simulink model "dynamics"  (R2022a)
settings: Solver=VariableStepAuto  StartTime=0.0  StopTime=10.0  RelTol=1e-3
undefined symbols (not defined in the file): b, g, h, I, J, K, L, m, R, Res
libraries: slpidlib x3
settings Model: Creator=daixingze  LastModifiedBy=xngzdai
settings SolverCC: AlgebraicLoopSolver=TrustRegion
settings DebuggingCC: UnconnectedInputMsg=warning  UnconnectedOutputMsg=warning  UnconnectedLineMsg=warning  SFMachineParentedDataDiag=warning

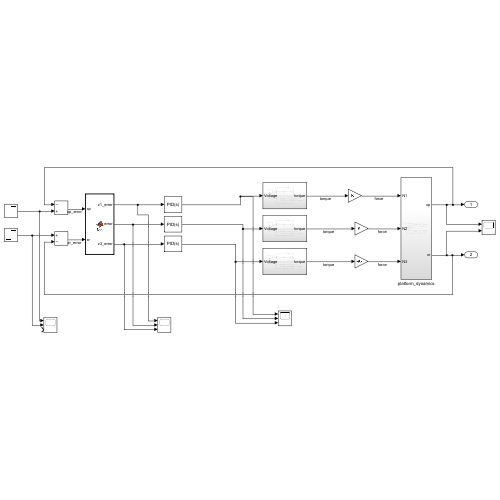
[thumbnail: Simulink's stored preview of the top-level diagram]
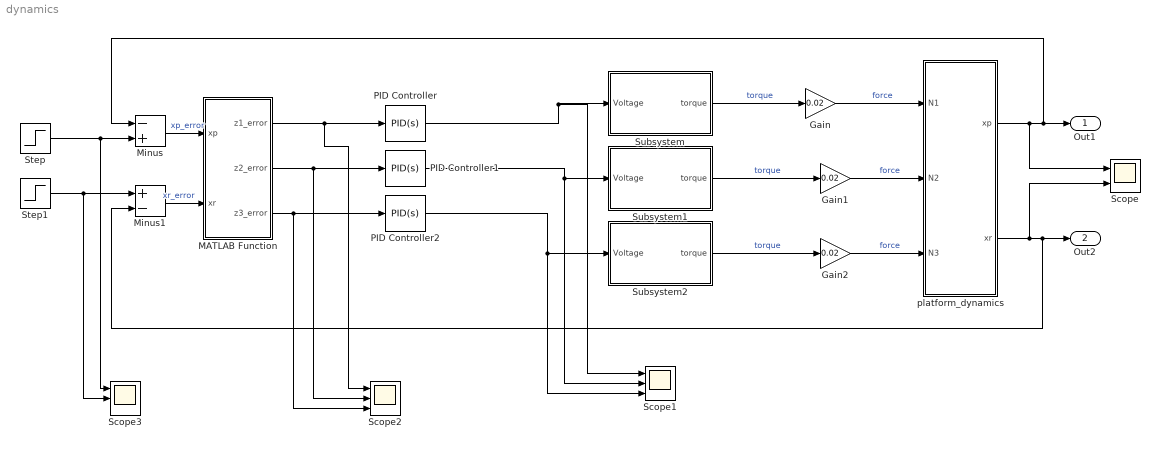
== system dynamics ==
  Gain : Gain  Gain=0.02
  Gain1 : Gain  Gain=0.02
  Gain2 : Gain  Gain=0.02
  MATLAB Function : MATLAB Function  TreatAsAtomicUnit=on
  Minus : Sum  Inputs=-+
  Minus1 : Sum  Inputs=+-
  PID Controller : slpidlib/PID Controller  Controller=PID  Form=Parallel  TimeDomain=Continuous-time  UseExternalTs=off  SampleTime=-1  IntegratorMethod=Forward Euler  FilterMethod=Forward Euler  ControllerParametersSource=internal  P=0.0002  I=0  UseKiTs=off  D=0.0000005  N=100  UseFilter=on  TunerSelectOption=Transfer Function Based (PID Tuner App)  InitialConditionSource=internal  InitialConditionForIntegrator=0  InitialConditionForFilter=0  DifferentiatorICPrevScaledInput=0  ExternalReset=none  TrackingMode=off  Kt=1  LimitOutput=off  SatLimitsSource=internal  UpperSaturationLimit=inf  LowerSaturationLimit=-inf  LinearizeAsGain=on  AntiWindupMode=none  Kb=1  POutMin=[]  POutMax=[]  IOutMin=[]  IOutMax=[]  DOutMin=[]  DOutMax=[]  NOutMin=[]  NOutMax=[]  SumOutMin=[]  SumOutMax=[]  SaturationOutMin=[]  SaturationOutMax=[]  PParamMin=[]  PParamMax=[]  IParamMin=[]  IParamMax=[]  DParamMin=[]  DParamMax=[]  NParamMin=[]  NParamMax=[]  KbParamMin=[]  KbParamMax=[]  KtParamMin=[]  KtParamMax=[]  KbOutMin=[]  KbOutMax=[]  KtOutMin=[]  KtOutMax=[]  IntegratorOutMin=[]  IntegratorOutMax=[]  FilterOutMin=[]  FilterOutMax=[]  SumI1OutMin=[]  SumI1OutMax=[]  SumI2OutMin=[]  SumI2OutMax=[]  SumI3OutMin=[]  SumI3OutMax=[]  SumI4OutMin=[]  SumI4OutMax=[]  SumDOutMin=[]  SumDOutMax=[]  DifferentiatorOutMin=[]  DifferentiatorOutMax=[]  FilterDiffOutCoefMin=[]  FilterDiffOutCoefMax=[]  ReciprocalOutMin=[]  ReciprocalOutMax=[]  SumDenOutMin=[]  SumDenOutMax=[]  SumNumOutMin=[]  SumNumOutMax=[]  DivideOutMin=[]  DivideOutMax=[]  UdiffTsProdOutMin=[]  UdiffTsProdOutMax=[]  NTsProdOutMin=[]  NTsProdOutMax=[]  UintegralTsProdOutMin=[]  UintegralTsProdOutMax=[]  UngainTsProdOutMin=[]  UngainTsProdOutMax=[]  IntegratorContinuousStateAttributes=''  IntegratorStateMustResolveToSignalObject=off  IntegratorRTWStateStorageClass=Auto  FilterContinuousStateAttributes=''  FilterStateMustResolveToSignalObject=off  FilterRTWStateStorageClass=Auto  ParallelPVariant=InternalParameters  IdealPVariant=Disabled  IVariant=InternalParameters  DVariant=InternalParameters  IntegratorVariant=Continuous  SatVariant=Disabled  AWVariant=Passthrough  PCopyVariant=Disabled  TRVariant=Disabled  FdbkBlocksVariant=Forward  IdealPFdbkVariant=Disabled  SatFdbkVariant=Disabled  DerivativeFilterVariant=ContFilter  NVariant=InternalParameters  NCopyVariant=Disabled  FilterICVariant=InternalICsFilter  IntegratorICVariant=InternalICs  ExternalResetVariant=Disabled  TRSumVariant=Passthrough  SumFdbkVariant=Disabled  SumVariant=Sum_PID  TsampFilterVariant=InternalTs  TsampNgainVariant=Passthrough  TsampIntegralVariant=Passthrough  ExternalSaturationOutDataTypeStr=Inherit: Same as second input  aMode=0
  PID Controller1 : slpidlib/PID Controller  Controller=PID  Form=Parallel  TimeDomain=Continuous-time  UseExternalTs=off  SampleTime=-1  IntegratorMethod=Forward Euler  FilterMethod=Forward Euler  ControllerParametersSource=internal  P=0.0002  I=0  UseKiTs=off  D=0.0000005  N=100  UseFilter=on  TunerSelectOption=Transfer Function Based (PID Tuner App)  InitialConditionSource=internal  InitialConditionForIntegrator=0  InitialConditionForFilter=0  DifferentiatorICPrevScaledInput=0  ExternalReset=none  TrackingMode=off  Kt=1  LimitOutput=off  SatLimitsSource=internal  UpperSaturationLimit=inf  LowerSaturationLimit=-inf  LinearizeAsGain=on  AntiWindupMode=none  Kb=1  POutMin=[]  POutMax=[]  IOutMin=[]  IOutMax=[]  DOutMin=[]  DOutMax=[]  NOutMin=[]  NOutMax=[]  SumOutMin=[]  SumOutMax=[]  SaturationOutMin=[]  SaturationOutMax=[]  PParamMin=[]  PParamMax=[]  IParamMin=[]  IParamMax=[]  DParamMin=[]  DParamMax=[]  NParamMin=[]  NParamMax=[]  KbParamMin=[]  KbParamMax=[]  KtParamMin=[]  KtParamMax=[]  KbOutMin=[]  KbOutMax=[]  KtOutMin=[]  KtOutMax=[]  IntegratorOutMin=[]  IntegratorOutMax=[]  FilterOutMin=[]  FilterOutMax=[]  SumI1OutMin=[]  SumI1OutMax=[]  SumI2OutMin=[]  SumI2OutMax=[]  SumI3OutMin=[]  SumI3OutMax=[]  SumI4OutMin=[]  SumI4OutMax=[]  SumDOutMin=[]  SumDOutMax=[]  DifferentiatorOutMin=[]  DifferentiatorOutMax=[]  FilterDiffOutCoefMin=[]  FilterDiffOutCoefMax=[]  ReciprocalOutMin=[]  ReciprocalOutMax=[]  SumDenOutMin=[]  SumDenOutMax=[]  SumNumOutMin=[]  SumNumOutMax=[]  DivideOutMin=[]  DivideOutMax=[]  UdiffTsProdOutMin=[]  UdiffTsProdOutMax=[]  NTsProdOutMin=[]  NTsProdOutMax=[]  UintegralTsProdOutMin=[]  UintegralTsProdOutMax=[]  UngainTsProdOutMin=[]  UngainTsProdOutMax=[]  IntegratorContinuousStateAttributes=''  IntegratorStateMustResolveToSignalObject=off  IntegratorRTWStateStorageClass=Auto  FilterContinuousStateAttributes=''  FilterStateMustResolveToSignalObject=off  FilterRTWStateStorageClass=Auto  ParallelPVariant=InternalParameters  IdealPVariant=Disabled  IVariant=InternalParameters  DVariant=InternalParameters  IntegratorVariant=Continuous  SatVariant=Disabled  AWVariant=Passthrough  PCopyVariant=Disabled  TRVariant=Disabled  FdbkBlocksVariant=Forward  IdealPFdbkVariant=Disabled  SatFdbkVariant=Disabled  DerivativeFilterVariant=ContFilter  NVariant=InternalParameters  NCopyVariant=Disabled  FilterICVariant=InternalICsFilter  IntegratorICVariant=InternalICs  ExternalResetVariant=Disabled  TRSumVariant=Passthrough  SumFdbkVariant=Disabled  SumVariant=Sum_PID  TsampFilterVariant=InternalTs  TsampNgainVariant=Passthrough  TsampIntegralVariant=Passthrough  ExternalSaturationOutDataTypeStr=Inherit: Same as second input  aMode=0
  PID Controller2 : slpidlib/PID Controller  Controller=PID  Form=Parallel  TimeDomain=Continuous-time  UseExternalTs=off  SampleTime=-1  IntegratorMethod=Forward Euler  FilterMethod=Forward Euler  ControllerParametersSource=internal  P=0.0002  I=0  UseKiTs=off  D=0.0000005  N=100  UseFilter=on  TunerSelectOption=Transfer Function Based (PID Tuner App)  InitialConditionSource=internal  InitialConditionForIntegrator=0  InitialConditionForFilter=0  DifferentiatorICPrevScaledInput=0  ExternalReset=none  TrackingMode=off  Kt=1  LimitOutput=off  SatLimitsSource=internal  UpperSaturationLimit=inf  LowerSaturationLimit=-inf  LinearizeAsGain=on  AntiWindupMode=none  Kb=1  POutMin=[]  POutMax=[]  IOutMin=[]  IOutMax=[]  DOutMin=[]  DOutMax=[]  NOutMin=[]  NOutMax=[]  SumOutMin=[]  SumOutMax=[]  SaturationOutMin=[]  SaturationOutMax=[]  PParamMin=[]  PParamMax=[]  IParamMin=[]  IParamMax=[]  DParamMin=[]  DParamMax=[]  NParamMin=[]  NParamMax=[]  KbParamMin=[]  KbParamMax=[]  KtParamMin=[]  KtParamMax=[]  KbOutMin=[]  KbOutMax=[]  KtOutMin=[]  KtOutMax=[]  IntegratorOutMin=[]  IntegratorOutMax=[]  FilterOutMin=[]  FilterOutMax=[]  SumI1OutMin=[]  SumI1OutMax=[]  SumI2OutMin=[]  SumI2OutMax=[]  SumI3OutMin=[]  SumI3OutMax=[]  SumI4OutMin=[]  SumI4OutMax=[]  SumDOutMin=[]  SumDOutMax=[]  DifferentiatorOutMin=[]  DifferentiatorOutMax=[]  FilterDiffOutCoefMin=[]  FilterDiffOutCoefMax=[]  ReciprocalOutMin=[]  ReciprocalOutMax=[]  SumDenOutMin=[]  SumDenOutMax=[]  SumNumOutMin=[]  SumNumOutMax=[]  DivideOutMin=[]  DivideOutMax=[]  UdiffTsProdOutMin=[]  UdiffTsProdOutMax=[]  NTsProdOutMin=[]  NTsProdOutMax=[]  UintegralTsProdOutMin=[]  UintegralTsProdOutMax=[]  UngainTsProdOutMin=[]  UngainTsProdOutMax=[]  IntegratorContinuousStateAttributes=''  IntegratorStateMustResolveToSignalObject=off  IntegratorRTWStateStorageClass=Auto  FilterContinuousStateAttributes=''  FilterStateMustResolveToSignalObject=off  FilterRTWStateStorageClass=Auto  ParallelPVariant=InternalParameters  IdealPVariant=Disabled  IVariant=InternalParameters  DVariant=InternalParameters  IntegratorVariant=Continuous  SatVariant=Disabled  AWVariant=Passthrough  PCopyVariant=Disabled  TRVariant=Disabled  FdbkBlocksVariant=Forward  IdealPFdbkVariant=Disabled  SatFdbkVariant=Disabled  DerivativeFilterVariant=ContFilter  NVariant=InternalParameters  NCopyVariant=Disabled  FilterICVariant=InternalICsFilter  IntegratorICVariant=InternalICs  ExternalResetVariant=Disabled  TRSumVariant=Passthrough  SumFdbkVariant=Disabled  SumVariant=Sum_PID  TsampFilterVariant=InternalTs  TsampNgainVariant=Passthrough  TsampIntegralVariant=Passthrough  ExternalSaturationOutDataTypeStr=Inherit: Same as second input  aMode=0
  Scope : Scope  NumInputPorts=2
  Scope1 : Scope  NumInputPorts=3
  Scope2 : Scope  NumInputPorts=3
  Scope3 : Scope  NumInputPorts=3
  Step : Step  After=0.002  SampleTime=0
  Step1 : Step  After=0  SampleTime=0
  Subsystem : Subsystem
  Subsystem1 : Subsystem
  Subsystem2 : Subsystem
  platform_dynamics : Subsystem
  Out1 : Outport
  Out2 : Outport  Port=2
  wires:
  platform_dynamics/1(xp) -> Scope/1, Minus/1, Out1/1
  platform_dynamics/2(xr) -> Scope/2, Minus1/2, Out2/1
  PID Controller/1 -> Subsystem/1(Voltage), Scope1/1
  Subsystem/1(torque) -> Gain/1  "torque"
  Gain/1 -> platform_dynamics/1(N1)  "force"
  Gain1/1 -> platform_dynamics/2(N2)  "force"
  PID Controller1/1 -> Scope1/2, Subsystem1/1(Voltage)
  Subsystem1/1(torque) -> Gain1/1  "torque"
  Gain2/1 -> platform_dynamics/3(N3)  "force"
  PID Controller2/1 -> Scope1/3, Subsystem2/1(Voltage)
  Subsystem2/1(torque) -> Gain2/1  "torque"
  Step/1 -> Scope3/1, Minus/2
  Minus/1 -> MATLAB Function/1(xp)  "xp_error"
  Step1/1 -> Scope3/2, Minus1/1
  Minus1/1 -> MATLAB Function/2(xr)  "xr_error"
  MATLAB Function/1(z1_error) -> Scope2/1, PID Controller/1
  MATLAB Function/2(z2_error) -> Scope2/2, PID Controller1/1
  MATLAB Function/3(z3_error) -> Scope2/3, PID Controller2/1

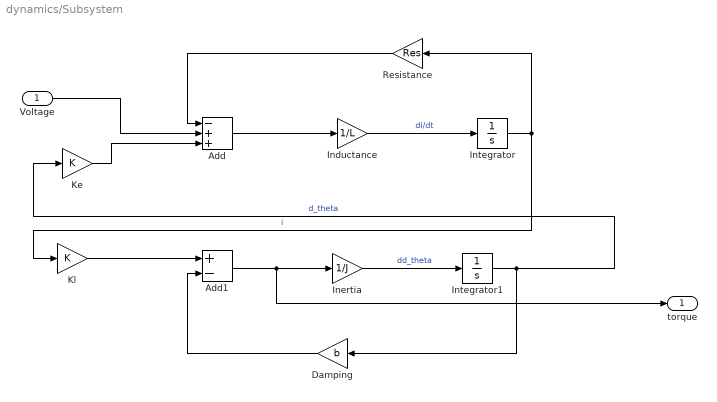
== system dynamics/Subsystem ==
  Voltage : Inport
  Add : Sum  Inputs=-++
  Add1 : Sum  Inputs=+-
  Damping : Gain  Gain=b
  Inductance : Gain  Gain=1/L
  Inertia : Gain  Gain=1/J
  Integrator : Integrator
  Integrator1 : Integrator
  Ke : Gain  Gain=K
  Kl : Gain  Gain=K
  Resistance : Gain  Gain=Res
  torque : Outport
  wires:
  Add/1 -> Inductance/1
  Inductance/1 -> Integrator/1  "di/dt"
  Voltage/1 -> Add/2
  Integrator1/1 -> Ke/1, Damping/1  "d_theta"
  Damping/1 -> Add1/2
  Kl/1 -> Add1/1
  Inertia/1 -> Integrator1/1  "dd_theta"
  Ke/1 -> Add/3
  Integrator/1 -> Kl/1, Resistance/1  "i"
  Resistance/1 -> Add/1
  Add1/1 -> torque/1, Inertia/1

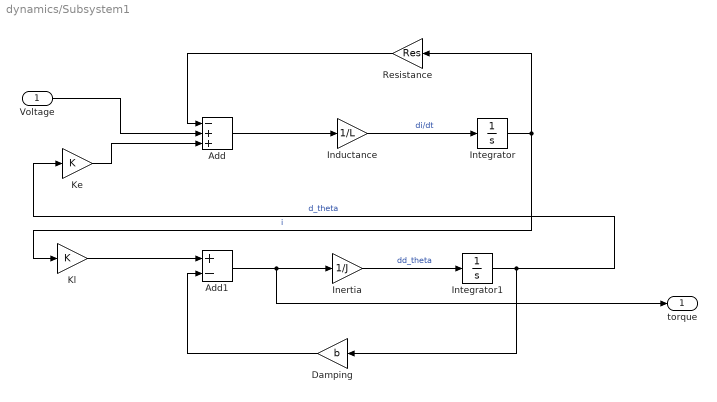
== system dynamics/Subsystem1 ==
  Voltage : Inport
  Add : Sum  Inputs=-++
  Add1 : Sum  Inputs=+-
  Damping : Gain  Gain=b
  Inductance : Gain  Gain=1/L
  Inertia : Gain  Gain=1/J
  Integrator : Integrator
  Integrator1 : Integrator
  Ke : Gain  Gain=K
  Kl : Gain  Gain=K
  Resistance : Gain  Gain=Res
  torque : Outport
  wires:
  Add/1 -> Inductance/1
  Inductance/1 -> Integrator/1  "di/dt"
  Voltage/1 -> Add/2
  Integrator1/1 -> Ke/1, Damping/1  "d_theta"
  Damping/1 -> Add1/2
  Kl/1 -> Add1/1
  Inertia/1 -> Integrator1/1  "dd_theta"
  Ke/1 -> Add/3
  Integrator/1 -> Kl/1, Resistance/1  "i"
  Resistance/1 -> Add/1
  Add1/1 -> torque/1, Inertia/1

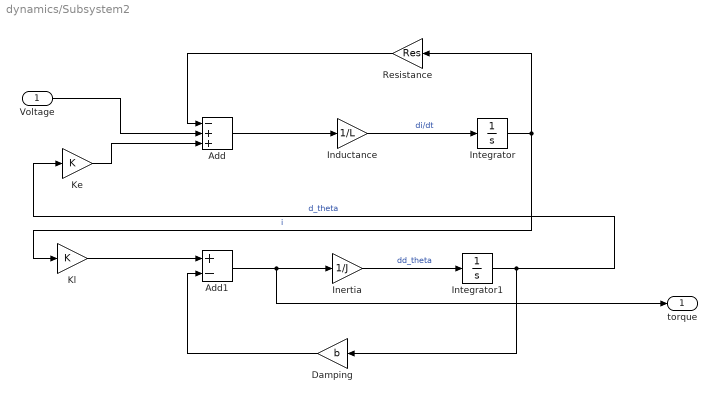
== system dynamics/Subsystem2 ==
  Voltage : Inport
  Add : Sum  Inputs=-++
  Add1 : Sum  Inputs=+-
  Damping : Gain  Gain=b
  Inductance : Gain  Gain=1/L
  Inertia : Gain  Gain=1/J
  Integrator : Integrator
  Integrator1 : Integrator
  Ke : Gain  Gain=K
  Kl : Gain  Gain=K
  Resistance : Gain  Gain=Res
  torque : Outport
  wires:
  Add/1 -> Inductance/1
  Inductance/1 -> Integrator/1  "di/dt"
  Voltage/1 -> Add/2
  Integrator1/1 -> Ke/1, Damping/1  "d_theta"
  Damping/1 -> Add1/2
  Kl/1 -> Add1/1
  Inertia/1 -> Integrator1/1  "dd_theta"
  Ke/1 -> Add/3
  Integrator/1 -> Kl/1, Resistance/1  "i"
  Resistance/1 -> Add/1
  Add1/1 -> torque/1, Inertia/1

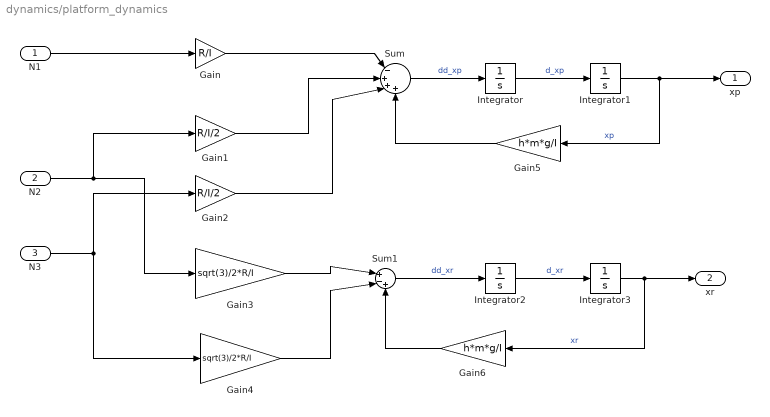
== system dynamics/platform_dynamics ==
  N1 : Inport
  N2 : Inport  Port=2
  N3 : Inport  Port=3
  Gain : Gain  Gain=R/I
  Gain1 : Gain  Gain=R/I/2
  Gain2 : Gain  Gain=R/I/2
  Gain3 : Gain  Gain=sqrt(3)/2*R/I
  Gain4 : Gain  Gain=sqrt(3)/2*R/I
  Gain5 : Gain  Gain=h*m*g/I
  Gain6 : Gain  Gain=h*m*g/I
  Integrator{,1..3} (4 alike) : Integrator
  Sum : Sum  Inputs=|-+++
  Sum1 : Sum  Inputs=|+-+
  xp : Outport
  xr : Outport  Port=2
  wires:
  Gain1/1 -> Sum/2
  Gain3/1 -> Sum1/1
  Sum/1 -> Integrator/1  "dd_xp"
  Integrator2/1 -> Integrator3/1  "d_xr"
  Gain2/1 -> Sum/3
  N3/1 -> Gain4/1, Gain2/1
  N1/1 -> Gain/1
  Integrator3/1 -> xr/1, Gain6/1  "xr"
  Integrator1/1 -> xp/1, Gain5/1  "xp"
  Gain6/1 -> Sum1/3
  Integrator/1 -> Integrator1/1  "d_xp"
  N2/1 -> Gain3/1, Gain1/1
  Gain5/1 -> Sum/4
  Gain4/1 -> Sum1/2
  Sum1/1 -> Integrator2/1  "dd_xr"
  Gain/1 -> Sum/1

== matlab function dynamics/MATLAB Function ==
  data: xp input; z1_error output; xr input; z2_error output; z3_error output
function [z1_error, z2_error, z3_error] = fcn(xp, xr)
    R = 0.02;
    z1_error = R * sin(xr);
    z2_error = R * sin(xp); % need to change
    z3_error = R * sin(xp); % need to change
